simulink model "Ny_MPPT_Simulink"  (R2026a)
settings: Solver=VariableStepAuto
values from neighbouring files (symbols this model uses):
  a = 20    [MPPTRegulator.m]    (also in Ny_MPPTRegulator.m)
  ad = 1/(n*Vt)    (= 0.5)    [MPPTRegulator.m]    (also in Ny_MPPTRegulator.m = 1.04166666667)
  b = 40    [MPPTRegulator.m]    (also in Ny_MPPTRegulator.m)
  G_ref = 1/1000    (= 0.001)    [Ny_MPPTRegulator.m]
  I_0 = 1e-2    (= 0.01)    [MPPTRegulator.m]    (also in Ny_MPPTRegulator.m = 0.0001)
  I_L = 5    [MPPTRegulator.m]    (also in Ny_MPPTRegulator.m)
  K_i = 5    [MPPTRegulator.m]    (also in Ny_MPPTRegulator.m)
  K_P = 0.5    [MPPTRegulator.m]    (also in Ny_MPPTRegulator.m = 0.2)
  R_s = 10    [MPPTRegulator.m]    (also in Ny_MPPTRegulator.m = 0)
  R_sh_inv = 1/R_sh    (= 0.002)    [Ny_MPPTRegulator.m]
  tau = 10^(-5)    (= 1e-05)    [Ny_MPPTRegulator.m]
  V_MMP = 9    [MPPTRegulator.m]    (also in Ny_MPPTRegulator.m = 4.8)
settings Model: Creator=tryma  LastModifiedBy=tryma

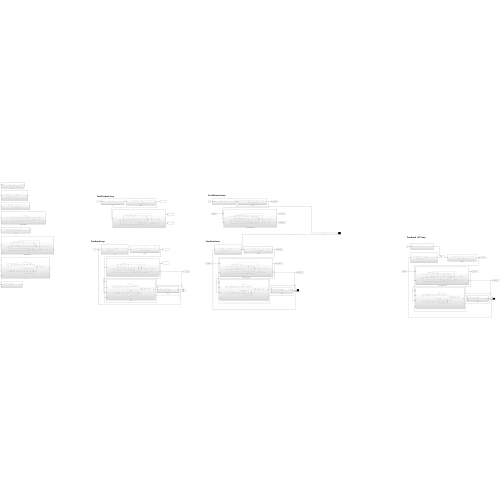
[thumbnail: Simulink's stored preview of the top-level diagram]
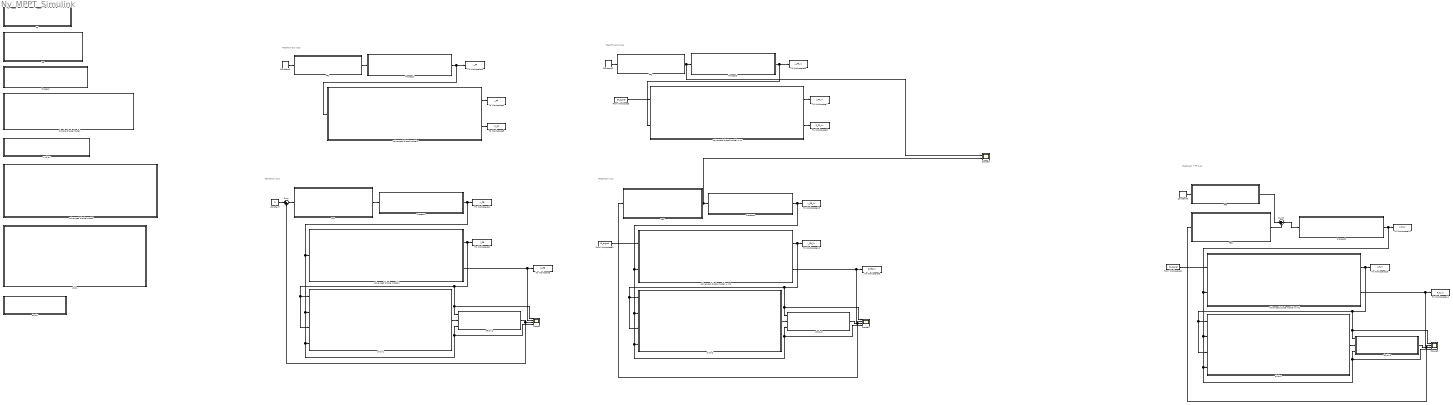
== system Ny_MPPT_Simulink ==
  note: Feedback loop
  note: FeedForward loop
  note: Feedback loop
  note: FeedForward loop
  note: Feedback + FF loop
  Advanced diode model : Subsystem
  Advanced diode model w.Irr : Subsystem
  Advanced diode model w.Irr1 : Subsystem
  Advanced diode model w.Irr2 : Subsystem
  Advanced diode model1 : Subsystem
  Advanced diode model2 : Subsystem
  Constant : Constant  Value=0
  Constant1 : Constant  Value=V_MMP
  Constant2 : Constant  Value=V_MMP
  Constant3 : Constant  Value=V_MMP
  FB : Subsystem
  FB1 : Subsystem
  FB2 : Subsystem
  FB3 : Subsystem
  FF : Subsystem
  FF1 : Subsystem
  FF2 : Subsystem
  FF3 : Subsystem
  From Workspace : FromWorkspace  VariableName=G_signal
  From Workspace1 : FromWorkspace  VariableName=G_signal
  From Workspace2 : FromWorkspace  VariableName=G_signal
  Prosess : Subsystem
  Prosess1 : Subsystem
  Prosess2 : Subsystem
  Prosess3 : Subsystem
  Prosess4 : Subsystem
  Prosess5 : Subsystem
  Scope : Scope  NumInputPorts=4
      settings: ActiveDisplayYMinimum=-14.542916422938951  ActiveDisplayYMaximum=94.785736263723578
  Scope1 : Scope  NumInputPorts=4
      settings: ActiveDisplayYMinimum=-14.542916422938951  ActiveDisplayYMaximum=94.785736263723578
  Scope2 : Scope  NumInputPorts=2
      settings: ActiveDisplayYMinimum=1.8337054871310838  ActiveDisplayYMaximum=10.320230649979909  DataLoggingVariableName=ScopeData2
  Scope3 : Scope  NumInputPorts=4
      settings: ActiveDisplayYMinimum=-14.542916422938951  ActiveDisplayYMaximum=94.785736263723578  DataLoggingVariableName=ScopeData3
  Simple Diode Model : Subsystem
  Sum : Sum  Inputs=|++
  Sum1 : Sum  Inputs=|++
  To Workspace : ToWorkspace  VariableName=P_FB  SaveFormat=Timeseries  SampleTime=-1
  To Workspace1 : ToWorkspace  VariableName=v_FB  SaveFormat=Timeseries  SampleTime=-1
  To Workspace10 : ToWorkspace  VariableName=v_FB_irr  SaveFormat=Timeseries  SampleTime=-1
  To Workspace11 : ToWorkspace  VariableName=i_FB_irr  SaveFormat=Timeseries  SampleTime=-1
  To Workspace12 : ToWorkspace  VariableName=v_F_irr  SaveFormat=Timeseries  SampleTime=-1
  To Workspace13 : ToWorkspace  VariableName=i_F_irr  SaveFormat=Timeseries  SampleTime=-1
  To Workspace14 : ToWorkspace  VariableName=P_F_irr  SaveFormat=Timeseries  SampleTime=-1
  To Workspace2 : ToWorkspace  VariableName=i_FB  SaveFormat=Timeseries  SampleTime=-1
  To Workspace3 : ToWorkspace  VariableName=v_FF  SaveFormat=Timeseries  SampleTime=-1
  To Workspace4 : ToWorkspace  VariableName=i_FF  SaveFormat=Timeseries  SampleTime=-1
  To Workspace5 : ToWorkspace  VariableName=P_FF  SaveFormat=Timeseries  SampleTime=-1
  To Workspace6 : ToWorkspace  VariableName=v_FF_irr  SaveFormat=Timeseries  SampleTime=-1
  To Workspace7 : ToWorkspace  VariableName=i_FF_irr  SaveFormat=Timeseries  SampleTime=-1
  To Workspace8 : ToWorkspace  VariableName=P_FF_irr  SaveFormat=Timeseries  SampleTime=-1
  To Workspace9 : ToWorkspace  VariableName=P_FB_irr  SaveFormat=Timeseries  SampleTime=-1
  dP/dv : Subsystem
  dP/dv1 : Subsystem
  dP/dv2 : Subsystem
  dP/dv3 : Subsystem
  di/dv : Subsystem
  di/dv1 : Subsystem
  di/dv2 : Subsystem
  di/dv3 : Subsystem
  v*di/dv : Subsystem
  wires:
  Constant/1 -> Sum/1
  Sum/1 -> FB1/1(e)
  FB1/1(u_fb) -> Prosess1/1(u)
  Prosess1/1(x) -> Scope/4, dP/dv1/3(x), di/dv1/4(x1), di/dv1/2(x), Advanced diode model1/1(x), To Workspace1/1  "v"
  Advanced diode model1/1(i) -> To Workspace2/1, Scope/1, dP/dv1/1(i), di/dv1/3(i1), di/dv1/1(i)  "i"
  di/dv1/1(di/dv) -> dP/dv1/2(di/dv)
  dP/dv1/1(dP/dv) -> Sum/2, Scope/3  "dP/dv"
  Advanced diode model1/2(P) -> Scope/2, To Workspace/1  "P"
  FF1/1(u_ff) -> Prosess2/1(u)
  Prosess2/1(x) -> To Workspace3/1, Advanced diode model2/1(x)  "v"
  Constant1/1 -> FF1/1(V_MMP)
  Advanced diode model2/1(i) -> To Workspace4/1
  Advanced diode model2/2(P) -> To Workspace5/1
  Advanced diode model w.Irr/2(P) -> To Workspace8/1
  Advanced diode model w.Irr/1(i) -> To Workspace7/1
  Constant2/1 -> FF2/1(V_MMP)
  Prosess3/1(x) -> Advanced diode model w.Irr/2(x), To Workspace6/1  "v"
  FF2/1(u_ff) -> Scope2/1, Prosess3/1(u)  "u_ff"
  From Workspace/1 -> Advanced diode model w.Irr/1(G)
  Advanced diode model w.Irr1/2(P) -> To Workspace9/1, Scope1/2  "P"
  dP/dv2/1(dP/dv) -> FB2/1(e), Scope1/3  "dP/dv"
  di/dv2/1(di/dv) -> dP/dv2/2(di/dv)
  Advanced diode model w.Irr1/1(i) -> di/dv2/1(i), di/dv2/3(i1), dP/dv2/1(i), Scope1/1, To Workspace11/1  "i"
  Prosess4/1(x) -> To Workspace10/1, Advanced diode model w.Irr1/2(x), di/dv2/2(x), di/dv2/4(x1), dP/dv2/3(x), Scope1/4  "v"
  FB2/1(u_fb) -> Scope2/2, Prosess4/1(u)  "u_fb"
  From Workspace1/1 -> Advanced diode model w.Irr1/1(G)
  From Workspace2/1 -> Advanced diode model w.Irr2/1(G)
  dP/dv3/1(dP/dv) -> FB3/1(e), Scope3/3  "dP/dv"
  Advanced diode model w.Irr2/2(P) -> To Workspace14/1, Scope3/2  "P"
  Advanced diode model w.Irr2/1(i) -> di/dv3/1(i), di/dv3/3(i1), dP/dv3/1(i), Scope3/1, To Workspace13/1  "i"
  Prosess5/1(x) -> To Workspace12/1, Advanced diode model w.Irr2/2(x), di/dv3/2(x), di/dv3/4(x1), dP/dv3/3(x), Scope3/4  "v"
  di/dv3/1(di/dv) -> dP/dv3/2(di/dv)
  Constant3/1 -> FF3/1(V_MMP)
  FF3/1(u_ff) -> Sum1/1  "u_ff"
  FB3/1(u_fb) -> Sum1/2  "u_fb"
  Sum1/1 -> Prosess5/1(u)  "u"

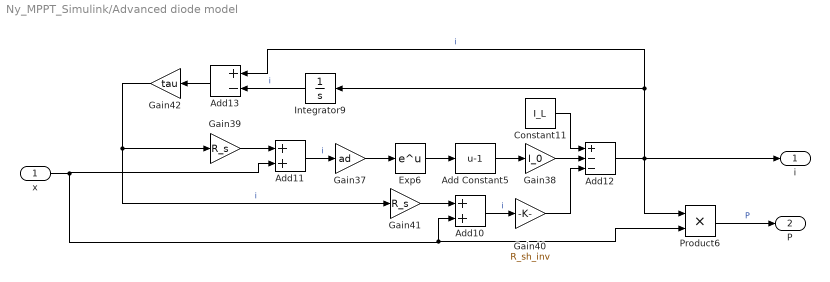
== system Ny_MPPT_Simulink/Advanced diode model ==
  x : Inport
  Add Constant5 : Bias  Bias=-1  SaturateOnIntegerOverflow=off
  Add10 : Sum
  Add11 : Sum
  Add12 : Sum  Inputs=+--
  Add13 : Sum  Inputs=+-
  Constant11 : Constant  Value=I_L
  Exp6 : Math
  Gain37 : Gain  Gain=ad
  Gain38 : Gain  Gain=I_0
  Gain39 : Gain  Gain=R_s
  Gain40 : Gain  Gain=R_sh_inv
  Gain41 : Gain  Gain=R_s
  Gain42 : Gain  Gain=tau
  Integrator9 : Integrator
  Product6 : Product
  i : Outport
  P : Outport  Port=2
  wires:
  Exp6/1 -> Add Constant5/1
  Gain40/1 -> Add12/3
  Gain39/1 -> Add11/1
  Gain42/1 -> Gain41/1, Gain39/1  "i"
  Add13/1 -> Gain42/1
  Add10/1 -> Gain40/1  "i"
  Add12/1 -> Product6/1, i/1, Add13/1, Integrator9/1  "i"
  Constant11/1 -> Add12/1
  Gain41/1 -> Add10/1
  Gain37/1 -> Exp6/1
  Add11/1 -> Gain37/1  "i"
  Add Constant5/1 -> Gain38/1
  x/1 -> Add11/2, Product6/2, Add10/2
  Gain38/1 -> Add12/2
  Integrator9/1 -> Add13/2  "i"
  Product6/1 -> P/1  "P"

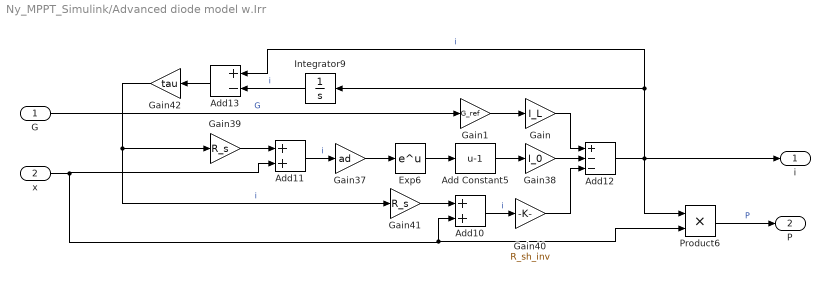
== system Ny_MPPT_Simulink/Advanced diode model w.Irr ==
  G : Inport
  x : Inport  Port=2
  Add Constant5 : Bias  Bias=-1  SaturateOnIntegerOverflow=off
  Add10 : Sum
  Add11 : Sum
  Add12 : Sum  Inputs=+--
  Add13 : Sum  Inputs=+-
  Exp6 : Math
  Gain : Gain  Gain=I_L
  Gain1 : Gain  Gain=G_ref
  Gain37 : Gain  Gain=ad
  Gain38 : Gain  Gain=I_0
  Gain39 : Gain  Gain=R_s
  Gain40 : Gain  Gain=R_sh_inv
  Gain41 : Gain  Gain=R_s
  Gain42 : Gain  Gain=tau
  Integrator9 : Integrator  InitialCondition=4
  Product6 : Product
  i : Outport
  P : Outport  Port=2
  wires:
  Product6/1 -> P/1  "P"
  Integrator9/1 -> Add13/2  "i"
  Gain38/1 -> Add12/2
  x/1 -> Add10/2, Product6/2, Add11/2
  Add Constant5/1 -> Gain38/1
  Add11/1 -> Gain37/1  "i"
  Gain37/1 -> Exp6/1
  Gain41/1 -> Add10/1
  Gain/1 -> Add12/1
  Add12/1 -> Integrator9/1, Add13/1, i/1, Product6/1  "i"
  Add10/1 -> Gain40/1  "i"
  Add13/1 -> Gain42/1
  Gain42/1 -> Gain39/1, Gain41/1  "i"
  Gain39/1 -> Add11/1
  Gain40/1 -> Add12/3
  Exp6/1 -> Add Constant5/1
  Gain1/1 -> Gain/1
  G/1 -> Gain1/1  "G"

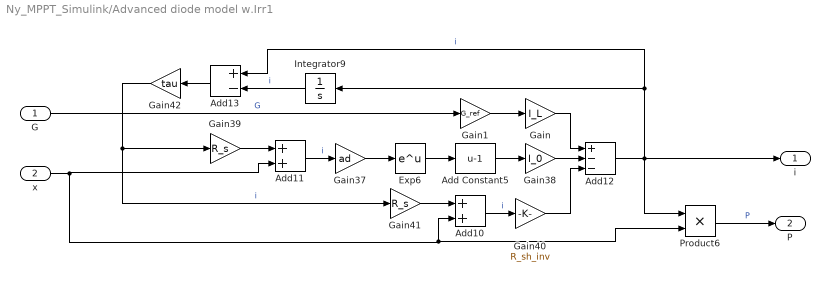
== system Ny_MPPT_Simulink/Advanced diode model w.Irr1 ==
  G : Inport
  x : Inport  Port=2
  Add Constant5 : Bias  Bias=-1  SaturateOnIntegerOverflow=off
  Add10 : Sum
  Add11 : Sum
  Add12 : Sum  Inputs=+--
  Add13 : Sum  Inputs=+-
  Exp6 : Math
  Gain : Gain  Gain=I_L
  Gain1 : Gain  Gain=G_ref
  Gain37 : Gain  Gain=ad
  Gain38 : Gain  Gain=I_0
  Gain39 : Gain  Gain=R_s
  Gain40 : Gain  Gain=R_sh_inv
  Gain41 : Gain  Gain=R_s
  Gain42 : Gain  Gain=tau
  Integrator9 : Integrator
  Product6 : Product
  i : Outport
  P : Outport  Port=2
  wires:
  G/1 -> Gain1/1  "G"
  Gain1/1 -> Gain/1
  Exp6/1 -> Add Constant5/1
  Gain40/1 -> Add12/3
  Gain39/1 -> Add11/1
  Gain42/1 -> Gain41/1, Gain39/1  "i"
  Add13/1 -> Gain42/1
  Add10/1 -> Gain40/1  "i"
  Add12/1 -> Product6/1, i/1, Add13/1, Integrator9/1  "i"
  Gain/1 -> Add12/1
  Gain41/1 -> Add10/1
  Gain37/1 -> Exp6/1
  Add11/1 -> Gain37/1  "i"
  Add Constant5/1 -> Gain38/1
  x/1 -> Add11/2, Product6/2, Add10/2
  Gain38/1 -> Add12/2
  Integrator9/1 -> Add13/2  "i"
  Product6/1 -> P/1  "P"

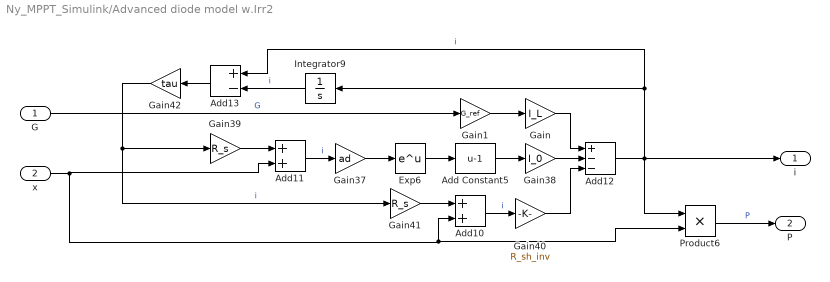
== system Ny_MPPT_Simulink/Advanced diode model w.Irr2 ==
  G : Inport
  x : Inport  Port=2
  Add Constant5 : Bias  Bias=-1  SaturateOnIntegerOverflow=off
  Add10 : Sum
  Add11 : Sum
  Add12 : Sum  Inputs=+--
  Add13 : Sum  Inputs=+-
  Exp6 : Math
  Gain : Gain  Gain=I_L
  Gain1 : Gain  Gain=G_ref
  Gain37 : Gain  Gain=ad
  Gain38 : Gain  Gain=I_0
  Gain39 : Gain  Gain=R_s
  Gain40 : Gain  Gain=R_sh_inv
  Gain41 : Gain  Gain=R_s
  Gain42 : Gain  Gain=tau
  Integrator9 : Integrator
  Product6 : Product
  i : Outport
  P : Outport  Port=2
  wires:
  G/1 -> Gain1/1  "G"
  Gain1/1 -> Gain/1
  Exp6/1 -> Add Constant5/1
  Gain40/1 -> Add12/3
  Gain39/1 -> Add11/1
  Gain42/1 -> Gain41/1, Gain39/1  "i"
  Add13/1 -> Gain42/1
  Add10/1 -> Gain40/1  "i"
  Add12/1 -> Product6/1, i/1, Add13/1, Integrator9/1  "i"
  Gain/1 -> Add12/1
  Gain41/1 -> Add10/1
  Gain37/1 -> Exp6/1
  Add11/1 -> Gain37/1  "i"
  Add Constant5/1 -> Gain38/1
  x/1 -> Add11/2, Product6/2, Add10/2
  Gain38/1 -> Add12/2
  Integrator9/1 -> Add13/2  "i"
  Product6/1 -> P/1  "P"

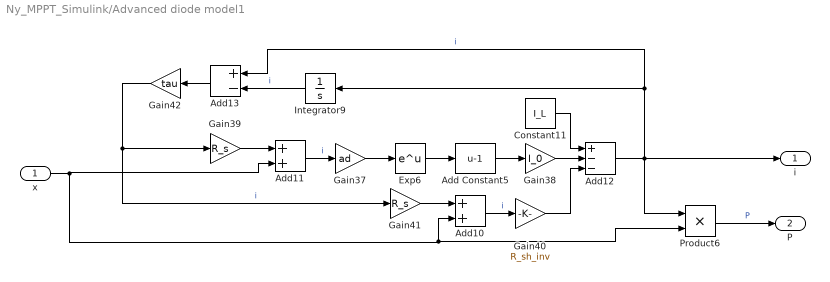
== system Ny_MPPT_Simulink/Advanced diode model1 ==
  x : Inport
  Add Constant5 : Bias  Bias=-1  SaturateOnIntegerOverflow=off
  Add10 : Sum
  Add11 : Sum
  Add12 : Sum  Inputs=+--
  Add13 : Sum  Inputs=+-
  Constant11 : Constant  Value=I_L
  Exp6 : Math
  Gain37 : Gain  Gain=ad
  Gain38 : Gain  Gain=I_0
  Gain39 : Gain  Gain=R_s
  Gain40 : Gain  Gain=R_sh_inv
  Gain41 : Gain  Gain=R_s
  Gain42 : Gain  Gain=tau
  Integrator9 : Integrator
  Product6 : Product
  i : Outport
  P : Outport  Port=2
  wires:
  Product6/1 -> P/1  "P"
  Integrator9/1 -> Add13/2  "i"
  Gain38/1 -> Add12/2
  x/1 -> Add10/2, Product6/2, Add11/2
  Add Constant5/1 -> Gain38/1
  Add11/1 -> Gain37/1  "i"
  Gain37/1 -> Exp6/1
  Gain41/1 -> Add10/1
  Constant11/1 -> Add12/1
  Add12/1 -> Integrator9/1, Add13/1, i/1, Product6/1  "i"
  Add10/1 -> Gain40/1  "i"
  Add13/1 -> Gain42/1
  Gain42/1 -> Gain39/1, Gain41/1  "i"
  Gain39/1 -> Add11/1
  Gain40/1 -> Add12/3
  Exp6/1 -> Add Constant5/1

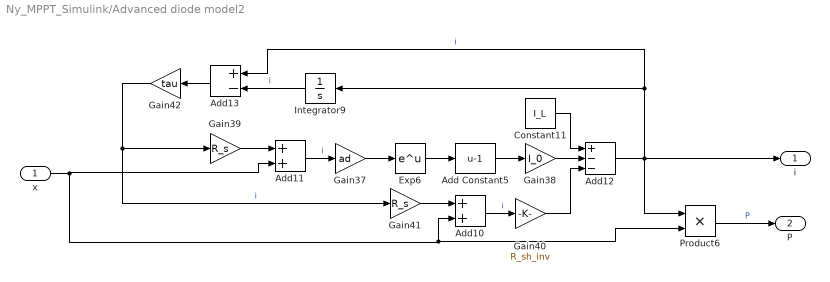
== system Ny_MPPT_Simulink/Advanced diode model2 ==
  x : Inport
  Add Constant5 : Bias  Bias=-1  SaturateOnIntegerOverflow=off
  Add10 : Sum
  Add11 : Sum
  Add12 : Sum  Inputs=+--
  Add13 : Sum  Inputs=+-
  Constant11 : Constant  Value=I_L
  Exp6 : Math
  Gain37 : Gain  Gain=ad
  Gain38 : Gain  Gain=I_0
  Gain39 : Gain  Gain=R_s
  Gain40 : Gain  Gain=R_sh_inv
  Gain41 : Gain  Gain=R_s
  Gain42 : Gain  Gain=tau
  Integrator9 : Integrator
  Product6 : Product
  i : Outport
  P : Outport  Port=2
  wires:
  Product6/1 -> P/1  "P"
  Integrator9/1 -> Add13/2  "i"
  Gain38/1 -> Add12/2
  x/1 -> Add10/2, Product6/2, Add11/2
  Add Constant5/1 -> Gain38/1
  Add11/1 -> Gain37/1  "i"
  Gain37/1 -> Exp6/1
  Gain41/1 -> Add10/1
  Constant11/1 -> Add12/1
  Add12/1 -> Integrator9/1, Add13/1, i/1, Product6/1  "i"
  Add10/1 -> Gain40/1  "i"
  Add13/1 -> Gain42/1
  Gain42/1 -> Gain39/1, Gain41/1  "i"
  Gain39/1 -> Add11/1
  Gain40/1 -> Add12/3
  Exp6/1 -> Add Constant5/1

== system Ny_MPPT_Simulink/FB ==
  e : Inport
  Add1 : Sum
  Gain6 : Gain  Gain=K_P
  Gain7 : Gain  Gain=K_i
  Integrator1 : Integrator
  u_fb : Outport
  wires:
  Gain6/1 -> Add1/1  "u_P"
  e/1 -> Gain7/1, Gain6/1
  Add1/1 -> u_fb/1  "u_fb"
  Integrator1/1 -> Add1/2  "u_I"
  Gain7/1 -> Integrator1/1

== system Ny_MPPT_Simulink/FB1 ==
  e : Inport
  Add1 : Sum
  Gain6 : Gain  Gain=K_P
  Gain7 : Gain  Gain=K_i
  Integrator1 : Integrator
  u_fb : Outport
  wires:
  Gain7/1 -> Integrator1/1
  Integrator1/1 -> Add1/2  "u_I"
  Add1/1 -> u_fb/1  "u_fb"
  e/1 -> Gain6/1, Gain7/1
  Gain6/1 -> Add1/1  "u_P"

== system Ny_MPPT_Simulink/FB2 ==
  e : Inport
  Add1 : Sum
  Gain6 : Gain  Gain=K_P
  Gain7 : Gain  Gain=K_i
  Integrator1 : Integrator
  u_fb : Outport
  wires:
  Gain6/1 -> Add1/1  "u_P"
  e/1 -> Gain7/1, Gain6/1
  Add1/1 -> u_fb/1  "u_fb"
  Integrator1/1 -> Add1/2  "u_I"
  Gain7/1 -> Integrator1/1

== system Ny_MPPT_Simulink/FB3 ==
  e : Inport
  Add1 : Sum
  Gain6 : Gain  Gain=K_P
  Gain7 : Gain  Gain=K_i
  Integrator1 : Integrator
  u_fb : Outport
  wires:
  Gain6/1 -> Add1/1  "u_P"
  e/1 -> Gain7/1, Gain6/1
  Add1/1 -> u_fb/1  "u_fb"
  Integrator1/1 -> Add1/2  "u_I"
  Gain7/1 -> Integrator1/1

== system Ny_MPPT_Simulink/FF ==
  V_MMP : Inport
  Gain4 : Gain  Gain=a
  Gain5 : Gain  Gain=1/b
  u_ff : Outport
  wires:
  Gain4/1 -> Gain5/1
  Gain5/1 -> u_ff/1  "u_ff"
  V_MMP/1 -> Gain4/1

== system Ny_MPPT_Simulink/FF1 ==
  V_MMP : Inport
  Gain4 : Gain  Gain=a
  Gain5 : Gain  Gain=1/b
  u_ff : Outport
  wires:
  V_MMP/1 -> Gain4/1
  Gain5/1 -> u_ff/1  "u_ff"
  Gain4/1 -> Gain5/1

== system Ny_MPPT_Simulink/FF2 ==
  V_MMP : Inport
  Gain4 : Gain  Gain=a
  Gain5 : Gain  Gain=1/b
  u_ff : Outport
  wires:
  Gain4/1 -> Gain5/1
  Gain5/1 -> u_ff/1  "u_ff"
  V_MMP/1 -> Gain4/1

== system Ny_MPPT_Simulink/FF3 ==
  V_MMP : Inport
  Gain4 : Gain  Gain=a
  Gain5 : Gain  Gain=1/b
  u_ff : Outport
  wires:
  V_MMP/1 -> Gain4/1
  Gain5/1 -> u_ff/1  "u_ff"
  Gain4/1 -> Gain5/1

== system Ny_MPPT_Simulink/Prosess ==
  u : Inport
  Gain : Gain  Gain=a
  Gain1 : Gain  Gain=b
  Integrator : Integrator
  Sum : Sum  Inputs=|+-
  x : Outport
  wires:
  Gain/1 -> Sum/2  "ax"
  Integrator/1 -> x/1, Gain/1  "x"
  u/1 -> Gain1/1
  Sum/1 -> Integrator/1  "x_dot"
  Gain1/1 -> Sum/1  "bu"

== system Ny_MPPT_Simulink/Prosess1 ==
  u : Inport
  Gain : Gain  Gain=a
  Gain1 : Gain  Gain=b
  Integrator : Integrator
  Sum : Sum  Inputs=|+-
  x : Outport
  wires:
  Gain1/1 -> Sum/1  "bu"
  Sum/1 -> Integrator/1  "x_dot"
  u/1 -> Gain1/1
  Integrator/1 -> Gain/1, x/1  "x"
  Gain/1 -> Sum/2  "ax"

== system Ny_MPPT_Simulink/Prosess2 ==
  u : Inport
  Gain : Gain  Gain=a
  Gain1 : Gain  Gain=b
  Integrator : Integrator
  Sum : Sum  Inputs=|+-
  x : Outport
  wires:
  Gain1/1 -> Sum/1  "bu"
  Sum/1 -> Integrator/1  "x_dot"
  u/1 -> Gain1/1
  Integrator/1 -> Gain/1, x/1  "x"
  Gain/1 -> Sum/2  "ax"

== system Ny_MPPT_Simulink/Prosess3 ==
  u : Inport
  Gain : Gain  Gain=a
  Gain1 : Gain  Gain=b
  Integrator : Integrator
  Sum : Sum  Inputs=|+-
  x : Outport
  wires:
  Gain/1 -> Sum/2  "ax"
  Integrator/1 -> x/1, Gain/1  "x"
  u/1 -> Gain1/1
  Sum/1 -> Integrator/1  "x_dot"
  Gain1/1 -> Sum/1  "bu"

== system Ny_MPPT_Simulink/Prosess4 ==
  u : Inport
  Gain : Gain  Gain=a
  Gain1 : Gain  Gain=b
  Integrator : Integrator
  Sum : Sum  Inputs=|+-
  x : Outport
  wires:
  Gain/1 -> Sum/2  "ax"
  Integrator/1 -> x/1, Gain/1  "x"
  u/1 -> Gain1/1
  Sum/1 -> Integrator/1  "x_dot"
  Gain1/1 -> Sum/1  "bu"

== system Ny_MPPT_Simulink/Prosess5 ==
  u : Inport
  Gain : Gain  Gain=a
  Gain1 : Gain  Gain=b
  Integrator : Integrator
  Sum : Sum  Inputs=|+-
  x : Outport
  wires:
  Gain/1 -> Sum/2  "ax"
  Integrator/1 -> x/1, Gain/1  "x"
  u/1 -> Gain1/1
  Sum/1 -> Integrator/1  "x_dot"
  Gain1/1 -> Sum/1  "bu"

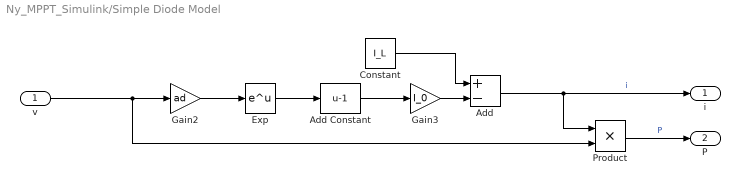
== system Ny_MPPT_Simulink/Simple Diode Model ==
  v : Inport
  Add : Sum  Inputs=+-
  Add Constant : Bias  Bias=-1  SaturateOnIntegerOverflow=off
  Constant : Constant  Value=I_L
  Exp : Math
  Gain2 : Gain  Gain=ad
  Gain3 : Gain  Gain=I_0
  Product : Product
  i : Outport
  P : Outport  Port=2
  wires:
  Gain2/1 -> Exp/1
  Constant/1 -> Add/1
  Add Constant/1 -> Gain3/1
  Add/1 -> i/1, Product/1  "i"
  Gain3/1 -> Add/2
  Product/1 -> P/1  "P"
  Exp/1 -> Add Constant/1
  v/1 -> Product/2, Gain2/1

== system Ny_MPPT_Simulink/dP//dv ==
  i : Inport
  di/dv : Inport  Port=2
  x : Inport  Port=3
  Add : Sum
  Product : Product
  dP/dv : Outport
  wires:
  di/dv/1 -> Product/1
  Product/1 -> Add/2
  x/1 -> Product/2
  i/1 -> Add/1
  Add/1 -> dP/dv/1  "dP/dv"

== system Ny_MPPT_Simulink/dP//dv1 ==
  i : Inport
  di/dv : Inport  Port=2
  x : Inport  Port=3
  Add : Sum
  Product : Product
  dP/dv : Outport
  wires:
  Add/1 -> dP/dv/1  "dP/dv"
  i/1 -> Add/1
  x/1 -> Product/2
  Product/1 -> Add/2
  di/dv/1 -> Product/1

== system Ny_MPPT_Simulink/dP//dv2 ==
  i : Inport
  di/dv : Inport  Port=2
  x : Inport  Port=3
  Add : Sum
  Product : Product
  dP/dv : Outport
  wires:
  di/dv/1 -> Product/1
  Product/1 -> Add/2
  x/1 -> Product/2
  i/1 -> Add/1
  Add/1 -> dP/dv/1  "dP/dv"

== system Ny_MPPT_Simulink/dP//dv3 ==
  i : Inport
  di/dv : Inport  Port=2
  x : Inport  Port=3
  Add : Sum
  Product : Product
  dP/dv : Outport
  wires:
  di/dv/1 -> Product/1
  Product/1 -> Add/2
  x/1 -> Product/2
  i/1 -> Add/1
  Add/1 -> dP/dv/1  "dP/dv"

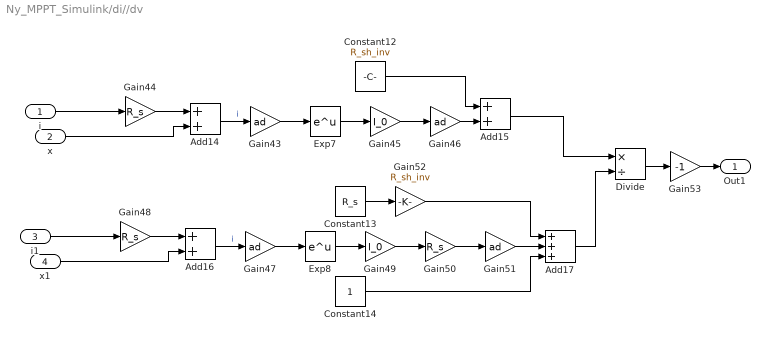
== system Ny_MPPT_Simulink/di//dv ==
  i : Inport
  x : Inport  Port=2
  i1 : Inport  Port=3
  x1 : Inport  Port=4
  Add14 : Sum
  Add15 : Sum
  Add16 : Sum
  Add17 : Sum  Inputs=+++
  Constant12 : Constant  Value=R_sh_inv
  Constant13 : Constant  Value=R_s
  Constant14 : Constant
  Divide : Product  Inputs=*/
  Exp7 : Math
  Exp8 : Math
  Gain{43,46..47,51} (4 alike) : Gain  Gain=ad
  Gain44 : Gain  Gain=R_s
  Gain45 : Gain  Gain=I_0
  Gain48 : Gain  Gain=R_s
  Gain49 : Gain  Gain=I_0
  Gain50 : Gain  Gain=R_s
  Gain52 : Gain  Gain=R_sh_inv
  Gain53 : Gain  Gain=-1
  Out1 : Outport
  wires:
  Constant12/1 -> Add15/1
  Gain43/1 -> Exp7/1
  Gain45/1 -> Gain46/1
  Exp8/1 -> Gain49/1
  Add14/1 -> Gain43/1  "i"
  Constant13/1 -> Gain52/1
  Gain49/1 -> Gain50/1
  Gain50/1 -> Gain51/1
  Gain47/1 -> Exp8/1
  Gain52/1 -> Add17/1
  x/1 -> Add14/2
  Gain46/1 -> Add15/2
  x1/1 -> Add16/2
  Add17/1 -> Divide/2
  Add15/1 -> Divide/1
  i1/1 -> Gain48/1
  Gain51/1 -> Add17/2
  Gain44/1 -> Add14/1
  Gain53/1 -> Out1/1
  Add16/1 -> Gain47/1  "i"
  Gain48/1 -> Add16/1
  Divide/1 -> Gain53/1
  Exp7/1 -> Gain45/1
  Constant14/1 -> Add17/3
  i/1 -> Gain44/1

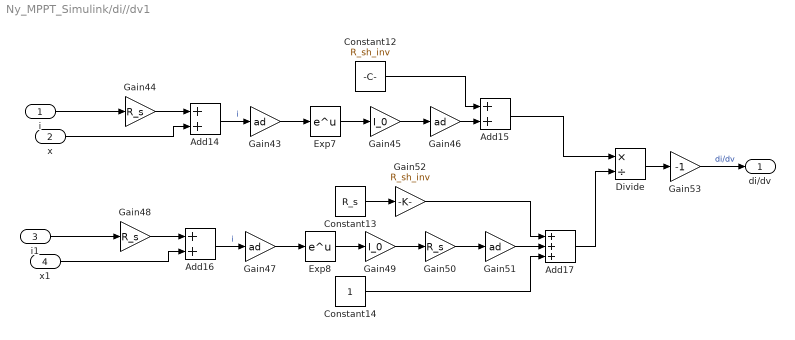
== system Ny_MPPT_Simulink/di//dv1 ==
  i : Inport
  x : Inport  Port=2
  i1 : Inport  Port=3
  x1 : Inport  Port=4
  Add14 : Sum
  Add15 : Sum
  Add16 : Sum
  Add17 : Sum  Inputs=+++
  Constant12 : Constant  Value=R_sh_inv
  Constant13 : Constant  Value=R_s
  Constant14 : Constant
  Divide : Product  Inputs=*/
  Exp7 : Math
  Exp8 : Math
  Gain{43,46..47,51} (4 alike) : Gain  Gain=ad
  Gain44 : Gain  Gain=R_s
  Gain45 : Gain  Gain=I_0
  Gain48 : Gain  Gain=R_s
  Gain49 : Gain  Gain=I_0
  Gain50 : Gain  Gain=R_s
  Gain52 : Gain  Gain=R_sh_inv
  Gain53 : Gain  Gain=-1
  di/dv : Outport
  wires:
  i/1 -> Gain44/1
  Constant14/1 -> Add17/3
  Exp7/1 -> Gain45/1
  Divide/1 -> Gain53/1
  Gain48/1 -> Add16/1
  Add16/1 -> Gain47/1  "i"
  Gain53/1 -> di/dv/1  "di/dv"
  Gain44/1 -> Add14/1
  Gain51/1 -> Add17/2
  i1/1 -> Gain48/1
  Add15/1 -> Divide/1
  Add17/1 -> Divide/2
  x1/1 -> Add16/2
  Gain46/1 -> Add15/2
  x/1 -> Add14/2
  Gain52/1 -> Add17/1
  Gain47/1 -> Exp8/1
  Gain50/1 -> Gain51/1
  Gain49/1 -> Gain50/1
  Constant13/1 -> Gain52/1
  Add14/1 -> Gain43/1  "i"
  Exp8/1 -> Gain49/1
  Gain45/1 -> Gain46/1
  Gain43/1 -> Exp7/1
  Constant12/1 -> Add15/1

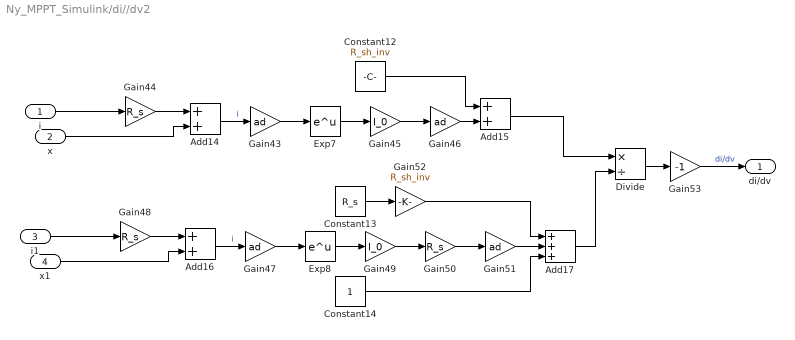
== system Ny_MPPT_Simulink/di//dv2 ==
  i : Inport
  x : Inport  Port=2
  i1 : Inport  Port=3
  x1 : Inport  Port=4
  Add14 : Sum
  Add15 : Sum
  Add16 : Sum
  Add17 : Sum  Inputs=+++
  Constant12 : Constant  Value=R_sh_inv
  Constant13 : Constant  Value=R_s
  Constant14 : Constant
  Divide : Product  Inputs=*/
  Exp7 : Math
  Exp8 : Math
  Gain{43,46..47,51} (4 alike) : Gain  Gain=ad
  Gain44 : Gain  Gain=R_s
  Gain45 : Gain  Gain=I_0
  Gain48 : Gain  Gain=R_s
  Gain49 : Gain  Gain=I_0
  Gain50 : Gain  Gain=R_s
  Gain52 : Gain  Gain=R_sh_inv
  Gain53 : Gain  Gain=-1
  di/dv : Outport
  wires:
  Constant12/1 -> Add15/1
  Gain43/1 -> Exp7/1
  Gain45/1 -> Gain46/1
  Exp8/1 -> Gain49/1
  Add14/1 -> Gain43/1  "i"
  Constant13/1 -> Gain52/1
  Gain49/1 -> Gain50/1
  Gain50/1 -> Gain51/1
  Gain47/1 -> Exp8/1
  Gain52/1 -> Add17/1
  x/1 -> Add14/2
  Gain46/1 -> Add15/2
  x1/1 -> Add16/2
  Add17/1 -> Divide/2
  Add15/1 -> Divide/1
  i1/1 -> Gain48/1
  Gain51/1 -> Add17/2
  Gain44/1 -> Add14/1
  Gain53/1 -> di/dv/1  "di/dv"
  Add16/1 -> Gain47/1  "i"
  Gain48/1 -> Add16/1
  Divide/1 -> Gain53/1
  Exp7/1 -> Gain45/1
  Constant14/1 -> Add17/3
  i/1 -> Gain44/1

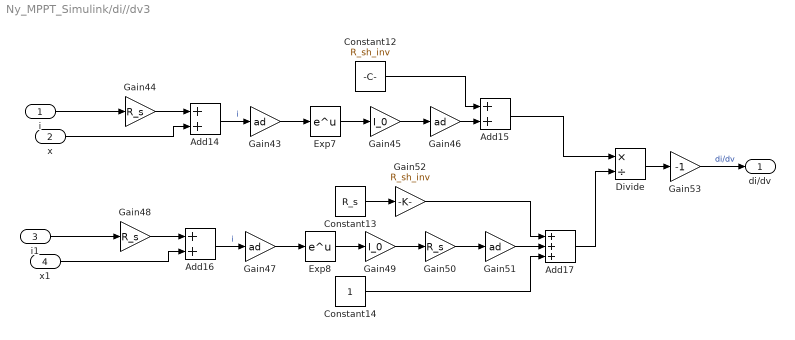
== system Ny_MPPT_Simulink/di//dv3 ==
  i : Inport
  x : Inport  Port=2
  i1 : Inport  Port=3
  x1 : Inport  Port=4
  Add14 : Sum
  Add15 : Sum
  Add16 : Sum
  Add17 : Sum  Inputs=+++
  Constant12 : Constant  Value=R_sh_inv
  Constant13 : Constant  Value=R_s
  Constant14 : Constant
  Divide : Product  Inputs=*/
  Exp7 : Math
  Exp8 : Math
  Gain{43,46..47,51} (4 alike) : Gain  Gain=ad
  Gain44 : Gain  Gain=R_s
  Gain45 : Gain  Gain=I_0
  Gain48 : Gain  Gain=R_s
  Gain49 : Gain  Gain=I_0
  Gain50 : Gain  Gain=R_s
  Gain52 : Gain  Gain=R_sh_inv
  Gain53 : Gain  Gain=-1
  di/dv : Outport
  wires:
  Constant12/1 -> Add15/1
  Gain43/1 -> Exp7/1
  Gain45/1 -> Gain46/1
  Exp8/1 -> Gain49/1
  Add14/1 -> Gain43/1  "i"
  Constant13/1 -> Gain52/1
  Gain49/1 -> Gain50/1
  Gain50/1 -> Gain51/1
  Gain47/1 -> Exp8/1
  Gain52/1 -> Add17/1
  x/1 -> Add14/2
  Gain46/1 -> Add15/2
  x1/1 -> Add16/2
  Add17/1 -> Divide/2
  Add15/1 -> Divide/1
  i1/1 -> Gain48/1
  Gain51/1 -> Add17/2
  Gain44/1 -> Add14/1
  Gain53/1 -> di/dv/1  "di/dv"
  Add16/1 -> Gain47/1  "i"
  Gain48/1 -> Add16/1
  Divide/1 -> Gain53/1
  Exp7/1 -> Gain45/1
  Constant14/1 -> Add17/3
  i/1 -> Gain44/1

== system Ny_MPPT_Simulink/v*di//dv ==
  v : Inport
  Exp5 : Math
  Gain34 : Gain  Gain=I_0
  Gain35 : Gain  Gain=ad
  Gain36 : Gain  Gain=ad
  Product5 : Product
  v*di/dv : Outport
  wires:
  Product5/1 -> v*di/dv/1  "v*di/dv"
  Gain35/1 -> Product5/2
  v/1 -> Product5/1, Gain36/1
  Gain36/1 -> Exp5/1
  Gain34/1 -> Gain35/1
  Exp5/1 -> Gain34/1
